simulink model "V2"  (Simulink 10.3)
settings: Solver=VariableStepAuto  StartTime=0.0  StopTime=0.1  RelTol=1e-3
libraries: spsDiodeLib x8, spsVoltageMeasurementLib x7, spsPVArrayLib x6, spsGroundLib x3, spsCurrentMeasurementLib x2, simulink x2, spsSeriesRLCBranchLib x1, spspowerguiLib x1
settings Model: Creator=ADMIN  LastModifiedBy=Haris
settings SolverCC: AlgebraicLoopSolver=Auto
settings DataIOCC: SaveFormat=Dataset  SignalLoggingSaveFormat=Dataset  ReturnWorkspaceOutputs=on
settings OptimizationCC: ExpressionDepthLimit=128  LifeSpan=auto
settings DebuggingCC: UnderspecifiedInitializationDetection=Simplified  MergeDetectMultiDrivingBlocksExec=error  FcnCallInpInsideContextMsg=error  StateNameClashWarn=none  SFUnexpectedBacktrackingDiag=error  SFNoUnconditionalDefaultTransitionDiag=error  SFExecutionAtInitializationDiag=warning  SFMachineParentedDataDiag=error  ArithmeticOperatorsInVariantConditions=error
settings HardwareCC: ProdBitPerPointer=64  ProdBitPerSizeT=64  ProdBitPerPtrDiffT=64  ProdLargestAtomicFloat=Float  ProdIntDivRoundTo=Zero  ProdEndianess=LittleEndian  ProdWordSize=64  ProdHWDeviceType=Intel->x86-64 (Windows64)
settings ModelReferenceCC: PropagateSignalLabelsOutOfModel=on
settings SFSimCC: SimUseLocalCustomCode=on  CustomCodeUndefinedFunction=FilterOut
settings RTWCC: RTWUseLocalCustomCode=on
settings CodeAppCC: StateflowObjectComments=off
settings GRTTargetCC: TargetLangStandard=C99 (ISO)  CombineOutputUpdateFcns=on  GRTInterface=off
settings ConfigComp: CovMetricSettings=dwe  CovSaveCumulativeToWorkspaceVar=off  CovSaveSingleToWorkspaceVar=off  CovExternalEMLEnable=on

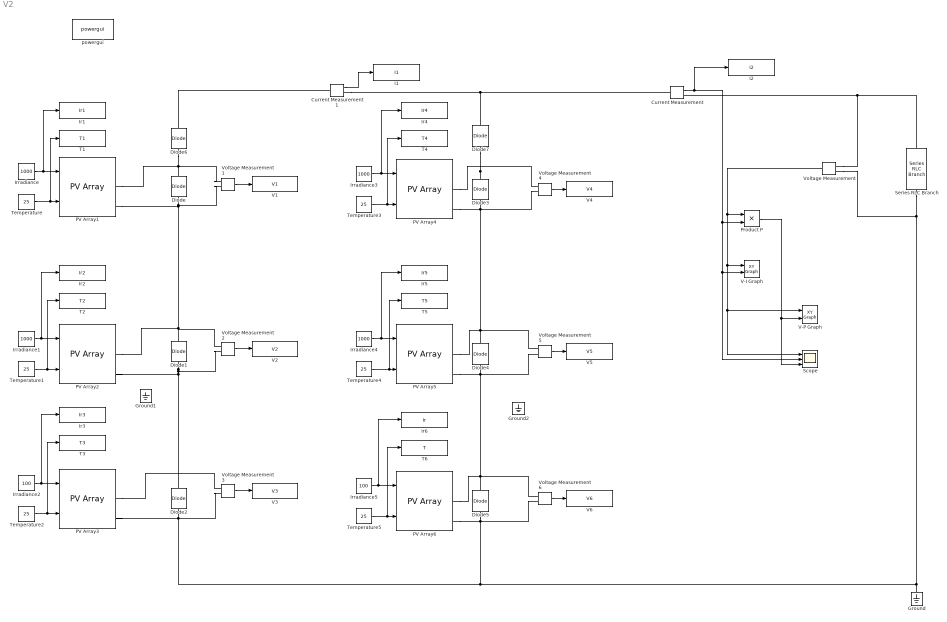
== system V2 ==
  Current Measurement : spsCurrentMeasurementLib/Current Measurement  PhasorSimulation=off  OutputType=Complex  PSBequivalent=0
  Current Measurement1 : spsCurrentMeasurementLib/Current Measurement  PhasorSimulation=off  OutputType=Complex  PSBequivalent=0
  Diode{,1..7} (8 alike) : spsDiodeLib/Diode  Ron=0.001  Lon=0  Vf=0.8  IC=0  UseSnubber=0  Rs=500  Cs=250e-9  Measurements=off
  Ground : spsGroundLib/Ground  LConnTagsString=a
  Ground1 : spsGroundLib/Ground  LConnTagsString=a
  Ground2 : spsGroundLib/Ground  LConnTagsString=a
  I1 : ToWorkspace  VariableName=I1  SampleTime=-1
      settings: Save2DSignal=2-D array (concatenate along first dimension)
  I2 : ToWorkspace  VariableName=I2  SampleTime=-1
      settings: Save2DSignal=2-D array (concatenate along first dimension)
  Ir1 : ToWorkspace  VariableName=Ir1  SampleTime=-1
      settings: Save2DSignal=2-D array (concatenate along first dimension)
  Ir2 : ToWorkspace  VariableName=Ir2  SampleTime=-1
      settings: Save2DSignal=2-D array (concatenate along first dimension)
  Ir3 : ToWorkspace  VariableName=Ir3  SampleTime=-1
      settings: Save2DSignal=2-D array (concatenate along first dimension)
  Ir4 : ToWorkspace  VariableName=Ir4  SampleTime=-1
      settings: Save2DSignal=2-D array (concatenate along first dimension)
  Ir5 : ToWorkspace  VariableName=Ir5  SampleTime=-1
      settings: Save2DSignal=2-D array (concatenate along first dimension)
  Ir6 : ToWorkspace  VariableName=Ir  SampleTime=-1
      settings: Save2DSignal=2-D array (concatenate along first dimension)
  Irradiance{,1,3..4} (4 alike) : Constant  Value=1000
  Irradiance2 : Constant  Value=100
  Irradiance5 : Constant  Value=100
  PV Array{1..6} (6 alike) : spsPVArrayLib/PV Array  Npar=1  Nser=1  PlotType=array @ 1000 W/m2 & specified temperatures  S_vec="[ 1000  500  100 ]"  Temp_C_vec="[ 45 25  ]"  ModuleName=Kyocera Solar KC200GT  PlotWhenSelected=off  Pm=200.143  Ncell=54  Voc=32.9  Isc=8.21  Vm=26.3  Im=7.61  beta_Voc_pc=-0.355  alpha_Isc_pc=0.06  beta_Voc=-0.11679  alpha_Isc=0.004926  IL=8.2288  I0=2.3234e-10  nI=0.97734  Rsh=150.6844  Rs=0.34484  RobustModel=off  RobustCellTemperature=313.3991  BAL=on  Tc=1e-6  Tfilter=5e-5
  Product P : Product
  Scope : Scope  NumInputPorts=3
  Series RLC Branch : spsSeriesRLCBranchLib/Series RLC Branch  LConnTagsString=__new0  RConnTagsString=__new0  BranchType=C  Resistance=1  Inductance=1e-3  SetiL0=off  InitialCurrent=0  Capacitance=1e-3  Setx0=off  InitialVoltage=0  Measurements=None
  T1 : ToWorkspace  VariableName=T1  SampleTime=-1
      settings: Save2DSignal=2-D array (concatenate along first dimension)
  T2 : ToWorkspace  VariableName=T2  SampleTime=-1
      settings: Save2DSignal=2-D array (concatenate along first dimension)
  T3 : ToWorkspace  VariableName=T3  SampleTime=-1
      settings: Save2DSignal=2-D array (concatenate along first dimension)
  T4 : ToWorkspace  VariableName=T4  SampleTime=-1
      settings: Save2DSignal=2-D array (concatenate along first dimension)
  T5 : ToWorkspace  VariableName=T5  SampleTime=-1
      settings: Save2DSignal=2-D array (concatenate along first dimension)
  T6 : ToWorkspace  VariableName=T  SampleTime=-1
      settings: Save2DSignal=2-D array (concatenate along first dimension)
  Temperature{,1..5} (6 alike) : Constant  Value=25
  V-I Graph : simulink/Sinks/XY Graph  xmin=0  xmax=100  ymin=1  ymax=18  st=-1
  V-P Graph : simulink/Sinks/XY Graph  xmin=0  xmax=100  ymin=0  ymax=1300  st=-1
  V1 : ToWorkspace  VariableName=V1  SampleTime=-1
      settings: Save2DSignal=2-D array (concatenate along first dimension)
  V2 : ToWorkspace  VariableName=V2  SampleTime=-1
      settings: Save2DSignal=2-D array (concatenate along first dimension)
  V3 : ToWorkspace  VariableName=V3  SampleTime=-1
      settings: Save2DSignal=2-D array (concatenate along first dimension)
  V4 : ToWorkspace  VariableName=V4  SampleTime=-1
      settings: Save2DSignal=2-D array (concatenate along first dimension)
  V5 : ToWorkspace  VariableName=V5  SampleTime=-1
      settings: Save2DSignal=2-D array (concatenate along first dimension)
  V6 : ToWorkspace  VariableName=V6  SampleTime=-1
      settings: Save2DSignal=2-D array (concatenate along first dimension)
  Voltage Measurement{,1..6} (7 alike) : spsVoltageMeasurementLib/Voltage Measurement  PhasorSimulation=off  OutputType=Complex  PSBequivalent=0
  powergui : spspowerguiLib/powergui  Priority=1  SimulationMode=Continuous  SampleTime=50e-6  frequency=60  Iterations=50  frequencyindice=0  Pbase=100e6  ErrMax=1e-4  UnitsV=kV  UnitsW=MW  buscounter=0  FunctionMessages=off  echomessages=off  EnableUseOfTLC=off  CurrentSourceSwitches=off  DisableSnubberDevices=off  DisableRonSwitches=off  DisableVfSwitches=off  DisplayEquations=off  AutomaticDiscreteSolvers=off  SolverType=Tustin/Backward Euler (TBE)  Interpol=off  ExternalGateDelay=off  methode=off  Ts=100  x0status=blocks  SPID=on  SwTol=0  HookPort=off  NonlinearTolerance=1e-4  nMaxIteration=100  ContinueOnMaxIteration=off  RestoreLinks=warning  ResistiveCurrentMeasurement=off  Frange=[0:2:500]  Ylog=off  Xlog=on  ShowGrid=off  save=off  variable=ZData  structure=0  ZoomFFT=off  StartTime=0.0  cycles=1  DisplayStyle=1  fundamental=60  FreqAxis=off  MaxFrequency=1000  frequencyindicesteady=1  RmsSteady=1  display=off
  wires:
  Product P/1 -> Scope/3, V-P Graph/2
  Voltage Measurement/1 -> Product P/1, Scope/1, V-P Graph/1, V-I Graph/1
  Temperature/1 -> T1/1, PV Array1/2
  Current Measurement/1 -> I2/1, Scope/2, V-I Graph/2, Product P/2
  Irradiance1/1 -> Ir2/1, PV Array2/1
  Irradiance4/1 -> Ir5/1, PV Array5/1
  Temperature4/1 -> T5/1, PV Array5/2
  Irradiance5/1 -> Ir6/1, PV Array6/1
  Irradiance3/1 -> Ir4/1, PV Array4/1
  Temperature2/1 -> T3/1, PV Array3/2
  Temperature5/1 -> T6/1, PV Array6/2
  Irradiance2/1 -> Ir3/1, PV Array3/1
  Temperature1/1 -> T2/1, PV Array2/2
  Irradiance/1 -> Ir1/1, PV Array1/1
  Temperature3/1 -> T4/1, PV Array4/2
  Voltage Measurement1/1 -> V1/1
  Current Measurement1/1 -> I1/1
  Voltage Measurement2/1 -> V2/1
  Voltage Measurement3/1 -> V3/1
  Voltage Measurement4/1 -> V4/1
  Voltage Measurement5/1 -> V5/1
  Voltage Measurement6/1 -> V6/1
  connections:
  Current Measurement/LConn1 -- Diode7/RConn1 -- Current Measurement1/RConn1
  PV Array5/RConn1 -- Voltage Measurement5/LConn1 -- Diode4/RConn1 -- Diode3/LConn1 -- Voltage Measurement4/LConn2 -- PV Array4/RConn2
  Voltage Measurement/LConn1 -- Series RLC Branch/LConn1 -- Current Measurement/RConn1
  Diode3/RConn1 -- Voltage Measurement4/LConn1 -- PV Array4/RConn1 -- Diode7/LConn1
  PV Array6/RConn1 -- Diode5/RConn1 -- Voltage Measurement6/LConn1 -- Diode4/LConn1 -- Voltage Measurement5/LConn2 -- PV Array5/RConn2
  PV Array1/RConn2 -- PV Array2/RConn1 -- Voltage Measurement2/LConn1 -- Diode1/RConn1 -- Voltage Measurement1/LConn2 -- Diode/LConn1
  Voltage Measurement/LConn2 -- Series RLC Branch/RConn1 -- Ground/LConn1 -- Voltage Measurement6/LConn2 -- PV Array6/RConn2 -- Diode5/LConn1 -- Voltage Measurement3/LConn2 -- PV Array3/RConn2 -- Diode2/LConn1
  Diode1/LConn1 -- PV Array3/RConn1 -- Diode2/RConn1 -- Voltage Measurement3/LConn1 -- PV Array2/RConn2 -- Voltage Measurement2/LConn2
  Voltage Measurement1/LConn1 -- PV Array1/RConn1 -- Diode6/LConn1 -- Diode/RConn1
  Current Measurement1/LConn1 -- Diode6/RConn1
